simulink model "vippip_win"  (Simulink 6.4)
settings: Solver=FixedStepDiscrete  StartTime=0.0  StopTime=inf  RelTol=1e-3
InitFcn:
  | initChan = str2num(get_param([bdroot(gcs) '/Control'],'pip_ch'));
model workspace: external: M-Code (data not in the file)
libraries: simulink x4, dspsigops x4, dspwin32 x3, vipgeotforms x2, dspswit3 x2, dspbuff3 x2, vipmisc x1, viptextngfix x1, vipsnks x1
CloseFcn:
  | clear initChan
settings Model: Creator=asharma  LastModifiedBy=Pr . Saddam&Ali
settings DataIOCC: SaveOutput=off  SaveTime=off
settings OptimizationCC: InlineInvariantSignals=on
settings DebuggingCC: StrictBusMsg=None

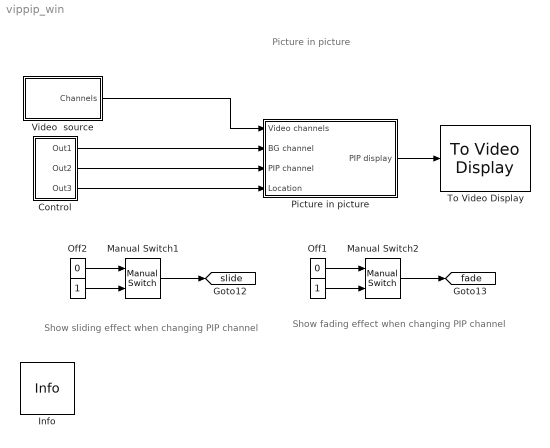
== system vippip_win ==
  note: Picture in picture
  note: Show sliding effect when
      | changing PIP channel
  note: Show fading effect  when
      |  changing PIP channel
  " " : Constant  Value=1  OutDataTypeMode=boolean  OutDataType=sfix(16)  ConRadixGroup=Use specified scaling  OutScaling=2^0  SampleTime=inf  FramePeriod=inf
  "   " : Constant  Value=1  OutDataTypeMode=boolean  OutDataType=sfix(16)  ConRadixGroup=Use specified scaling  OutScaling=2^0  SampleTime=inf  FramePeriod=inf
  Control : Subsystem  mask(Control){main_ch=1, pip_ch=2, piplocation=Lower left}
      mask prompts: main_ch "Main channel number"; pip_ch "PIP channel number"; piplocation "Location of PIP window"
      mask help: User this mask to control the channel choices and location of the picture in picture (PIP) window.
      mask init:
      | if (piplocation==1)
      |     quadLoc1= '[0 0]';
      | elseif (piplocation==2)
      |     quadLoc1 = '[0 80]';
      | elseif (piplocation==4)
      |     quadLoc1= '[60 80]';
      | else
      |     quadLoc1 = '[60 0]';
      | end
      | set_param([gcb '/Location of PIP video'], 'Value', quadLoc1);
      mask StyleString: popup(1|2|3),popup(1|2|3),popup(Upper left|Upper right|Lower left|Lower right)
      mask Display: disp('Control');
  Info : vipmisc/Info  SystemSampleTime=-1
  Manual Switch1 : simulink/Signal Routing/Manual Switch  SystemSampleTime=-1  sw=0  action=0
  Manual Switch2 : simulink/Signal Routing/Manual Switch  SystemSampleTime=-1  sw=0  action=0
  Off1 : Constant  Value=0  OutDataTypeMode=boolean  OutDataType=sfix(16)  ConRadixGroup=Use specified scaling  OutScaling=2^0  SampleTime=inf  FramePeriod=inf
  Off2 : Constant  Value=0  OutDataTypeMode=boolean  OutDataType=sfix(16)  ConRadixGroup=Use specified scaling  OutScaling=2^0  SampleTime=inf  FramePeriod=inf
  Picture in picture : Subsystem
  To Video Display : vipsnks/To Video Display  inputType=Intensity  OutputDevice=On-screen video monitor  fullScreen=off  videoWindowX=711  videoWindowY=334  saveWindowSize=off  videoWindowWidth=168  videoWindowHeight=147
  Video  source : Subsystem
  tag scope: fade=global, slide=global
  wires:
  Picture in picture/1(PIP display) -> To Video Display/1
  Off1/1 -> Manual Switch2/1
  "   "/1 -> Manual Switch2/2
  Manual Switch2/1 -> [fade]
  Off2/1 -> Manual Switch1/1
  " "/1 -> Manual Switch1/2
  Manual Switch1/1 -> [slide]
  Video  source/1(Channels) -> Picture in picture/1(Video channels)
  Control/1(Out1) -> Picture in picture/2(BG channel)
  Control/2(Out2) -> Picture in picture/3(PIP channel)
  Control/3(Out3) -> Picture in picture/4(Location)

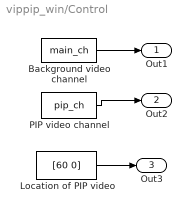
== system vippip_win/Control ==
  Background video channel : Constant  Value=main_ch  OutDataTypeMode=single  OutDataType=sfix(16)  ConRadixGroup=Use specified scaling  OutScaling=2^0  SampleTime=1/30  FramePeriod=inf
  Location of PIP video : Constant  Value=[60 0]  OutDataTypeMode=single  OutDataType=sfix(16)  ConRadixGroup=Use specified scaling  OutScaling=2^0  SampleTime=1/30  FramePeriod=inf
  PIP video channel : Constant  Value=pip_ch  OutDataTypeMode=single  OutDataType=sfix(16)  ConRadixGroup=Use specified scaling  OutScaling=2^0  SampleTime=1/30  FramePeriod=inf
  Out1 : Outport
  Out2 : Outport  Port=2
  Out3 : Outport  Port=3
  wires:
  Background video channel/1 -> Out1/1
  PIP video channel/1 -> Out2/1
  Location of PIP video/1 -> Out3/1

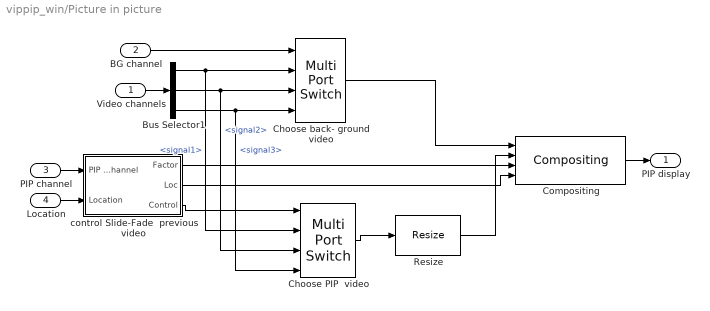
== system vippip_win/Picture in picture ==
  Video channels : Inport
  BG channel : Inport  Port=2
  PIP channel : Inport  Port=3
  Location : Inport  Port=4
  Bus Selector1 : BusSelector  OutputSignals=signal1,signal2,signal3
  Choose PIP  video : MultiPortSwitch  Inputs=3  InputSameDT=on
  Choose back- ground video : MultiPortSwitch  Inputs=3  InputSameDT=on
  Compositing : viptextngfix/Compositing  DialogController=vipDDGCreate  DialogControllerArgs=DataTag0  operation=Blend  bFacSrc=Input port  mFacSrc=Specify via dialog  bFactor=0.5  mFactor=1  source=Input port  coordinates=[0 0]  prodOutputMode=Binary point scaling  prodOutputWordLength=32  prodOutputFracLength=10  roundingMode=Floor  overflowMode=off
  Resize : vipgeotforms/Resize  DialogController=vipDDGCreate  DialogControllerArgs=DataTag1  specify=Output size as a percentage of input size  rfactor=50  outCols=25  outRows=25  outRowsCols=[60 80]  interp_method=Bilinear  antialias=on  prodOutputMode=Binary point scaling  prodOutputWordLength=32  prodOutputFracLength=10  roundingMode=Nearest  overflowMode=on
  control Slide-Fade  previous video : Subsystem
  PIP display : Outport
  wires:
  Choose PIP  video/1 -> Resize/1
  control Slide-Fade  previous video/3(Control) -> Choose PIP  video/1
  control Slide-Fade  previous video/2(Loc) -> Compositing/4
  control Slide-Fade  previous video/1(Factor) -> Compositing/3
  Choose back- ground video/1 -> Compositing/1
  Resize/1 -> Compositing/2
  Bus Selector1/1 -> Choose back- ground video/2, Choose PIP  video/2  "<signal1>"
  Bus Selector1/2 -> Choose back- ground video/3, Choose PIP  video/3  "<signal2>"
  Bus Selector1/3 -> Choose back- ground video/4, Choose PIP  video/4  "<signal3>"
  BG channel/1 -> Choose back- ground video/1
  Video channels/1 -> Bus Selector1/1
  Compositing/1 -> PIP display/1
  PIP channel/1 -> control Slide-Fade  previous video/1(PIP video channel)
  Location/1 -> control Slide-Fade  previous video/2(Location)

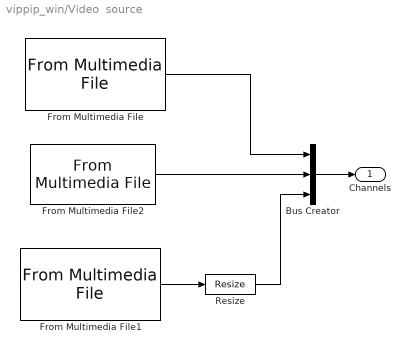
== system vippip_win/Video  source ==
  Bus Creator : BusCreator  Inputs=3
  From Multimedia File : dspwin32/From Multimedia File  DialogController=dspDDGCreate  DialogControllerArgs=DataTag2  inputFilename=cat_video.avi  loop=on  numPlays=inf  outputStreams=Video and audio  videoDataType=single  audioDataType=int16  inheritSampleTime=on  userDefinedSampleTime=1/30  noAudioOutput=off  isIntensityVideo=on  outputEOF=off
  From Multimedia File1 : dspwin32/From Multimedia File  DialogController=dspDDGCreate  DialogControllerArgs=DataTag3  inputFilename=shaky_car.avi  loop=on  numPlays=inf  outputStreams=Video and audio  videoDataType=single  audioDataType=int16  inheritSampleTime=on  userDefinedSampleTime=1/30  noAudioOutput=off  isIntensityVideo=on  outputEOF=off
  From Multimedia File2 : dspwin32/From Multimedia File  DialogController=dspDDGCreate  DialogControllerArgs=DataTag4  inputFilename=vipmen.avi  loop=on  numPlays=inf  outputStreams=Video and audio  videoDataType=single  audioDataType=int16  inheritSampleTime=on  userDefinedSampleTime=1/30  noAudioOutput=off  isIntensityVideo=on  outputEOF=off
  Resize : vipgeotforms/Resize  DialogController=vipDDGCreate  DialogControllerArgs=DataTag5  specify=Number of output rows and columns  rfactor=200  outCols=25  outRows=25  outRowsCols=[120 160]  interp_method=Bilinear  antialias=on  prodOutputMode=Binary point scaling  prodOutputWordLength=32  prodOutputFracLength=10  roundingMode=Nearest  overflowMode=on
  Channels : Outport
  wires:
  From Multimedia File1/1 -> Resize/1
  From Multimedia File/1 -> Bus Creator/1
  From Multimedia File2/1 -> Bus Creator/2
  Resize/1 -> Bus Creator/3
  Bus Creator/1 -> Channels/1

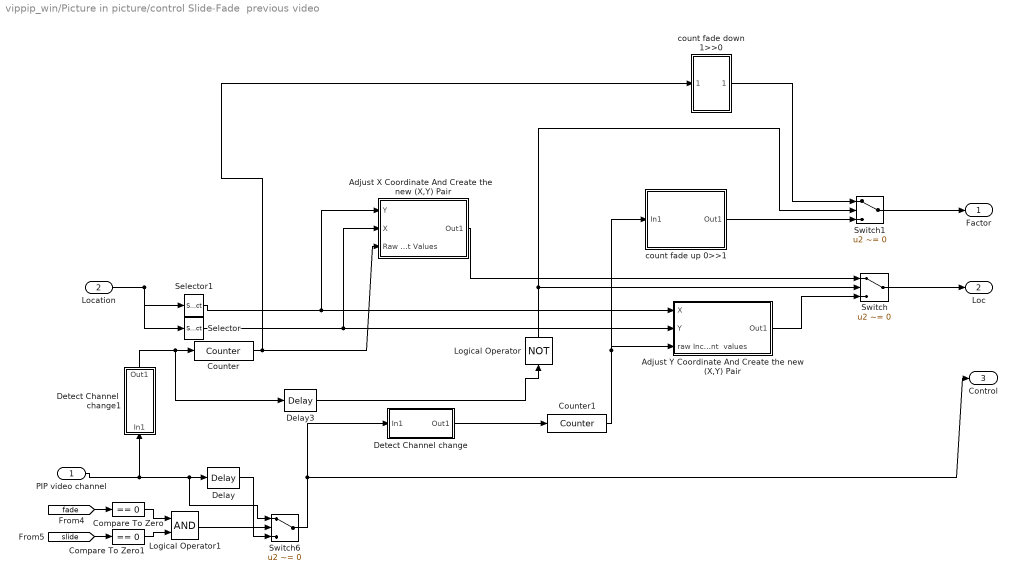
== system vippip_win/Picture in picture/control Slide-Fade  previous video ==
  PIP video channel : Inport
  Location : Inport  Port=2
  Adjust X Coordinate And Create the   new (X,Y) Pair : Subsystem
  Adjust Y Coordinate And Create the new (X,Y) Pair : Subsystem
  Compare To Zero : simulink/Logic and Bit Operations/Compare To Zero  SystemSampleTime=-1  relop===  LogicOutDataTypeMode=uint8  ZeroCross=off
  Compare To Zero1 : simulink/Logic and Bit Operations/Compare To Zero  SystemSampleTime=-1  relop===  LogicOutDataTypeMode=uint8  ZeroCross=off
  Counter : dspswit3/Counter  Direction=Up  CountEvent=Non-zero sample  CounterSize=User defined  MaxCount=31  InitialCount=0  Output=Count  HitValue=32  ResetInput=off  SamplesPerFrame=1  Ts=1/(30.0375)  CntDtype=single  HitDtype=Logical
  Counter1 : dspswit3/Counter  Direction=Up  CountEvent=Non-zero sample  CounterSize=User defined  MaxCount=31  InitialCount=0  Output=Count  HitValue=32  ResetInput=off  SamplesPerFrame=1  Ts=1/(30.0375)  CntDtype=single  HitDtype=Logical
  Delay : dspsigops/Delay  dly_unit=Samples  delay=32  ic_detail=on  dif_ic_for_ch=off  dif_ic_for_dly=off  ic=initChan  reset_popup=None
  Delay3 : dspsigops/Delay  dly_unit=Samples  delay=31  ic_detail=on  dif_ic_for_ch=off  dif_ic_for_dly=off  ic=initChan  reset_popup=None
  Detect Channel  change1 : Subsystem  Orientation=up
  Detect Channel change : Subsystem
  Logical Operator : Logic  Orientation=up  Operator=NOT  AllPortsSameDT=off  OutDataTypeMode=Boolean
  Logical Operator1 : Logic  AllPortsSameDT=off  OutDataTypeMode=Boolean
  Selector : Selector  Elements=2  InputPortWidth=2
  Selector1 : Selector  InputPortWidth=2
  Switch : Switch  Criteria=u2 ~= 0
  Switch1 : Switch  Criteria=u2 ~= 0
  Switch6 : Switch  Criteria=u2 ~= 0
  count fade down 1>>0 : Subsystem
  count fade up 0>>1 : Subsystem
  Factor : Outport
  Loc : Outport  Port=2
  Control : Outport  Port=3
  wires:
  Switch6/1 -> Control/1, Detect Channel change/1(In1)
  Delay/1 -> Switch6/3
  Logical Operator1/1 -> Switch6/2
  Compare To Zero1/1 -> Logical Operator1/2
  Compare To Zero/1 -> Logical Operator1/1
  [slide] -> Compare To Zero1/1
  [fade] -> Compare To Zero/1
  count fade up 0>>1/1(Out1) -> Switch1/3
  PIP video channel/1 -> Switch6/1, Delay/1, Detect Channel  change1/1(In1)
  Counter/1 -> count fade down 1>>0/1(In1), Adjust X Coordinate And Create the   new (X,Y) Pair/3(Raw Count Values)
  Selector1/1 -> Adjust Y Coordinate And Create the new (X,Y) Pair/1(X), Adjust X Coordinate And Create the   new (X,Y) Pair/1(Y)
  Location/1 -> Selector/1, Selector1/1
  Selector/1 -> Adjust Y Coordinate And Create the new (X,Y) Pair/2(Y), Adjust X Coordinate And Create the   new (X,Y) Pair/2(X)
  Detect Channel  change1/1(Out1) -> Counter/1, Delay3/1
  Detect Channel change/1(Out1) -> Counter1/1
  Counter1/1 -> count fade up 0>>1/1(In1), Adjust Y Coordinate And Create the new (X,Y) Pair/3(raw Increment  values)
  Adjust X Coordinate And Create the   new (X,Y) Pair/1(Out1) -> Switch/1
  Adjust Y Coordinate And Create the new (X,Y) Pair/1(Out1) -> Switch/3
  Switch/1 -> Loc/1
  Logical Operator/1 -> Switch/2, Switch1/2
  Delay3/1 -> Logical Operator/1
  count fade down 1>>0/1(Out1) -> Switch1/1
  Switch1/1 -> Factor/1

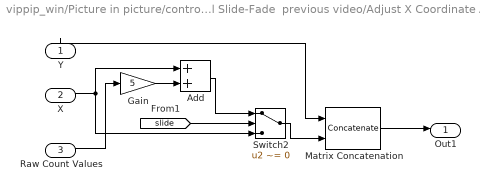
== system vippip_win/Picture in picture/control Slide-Fade  previous video/Adjust X Coordinate And Create the   new (X,Y) Pair ==
  Y : Inport  Orientation=up
  X : Inport  Port=2
  Raw Count Values : Inport  Port=3
  Add : Sum  OutScaling=2^-10
  Gain : Gain  Gain=5
  Matrix Concatenation : Concatenate  Mode=Horizontal matrix concatenation
  Switch2 : Switch  Criteria=u2 ~= 0
  Out1 : Outport
  wires:
  Switch2/1 -> Matrix Concatenation/2
  Add/1 -> Switch2/1
  [slide] -> Switch2/2
  Gain/1 -> Add/2
  Y/1 -> Matrix Concatenation/1
  X/1 -> Add/1, Switch2/3
  Raw Count Values/1 -> Gain/1
  Matrix Concatenation/1 -> Out1/1

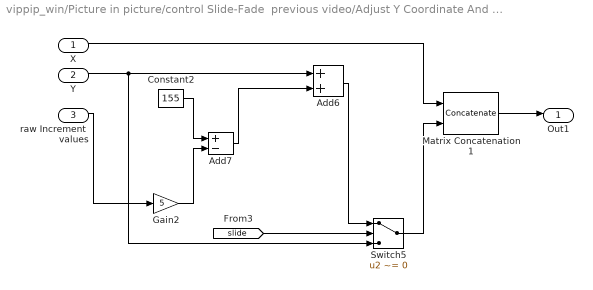
== system vippip_win/Picture in picture/control Slide-Fade  previous video/Adjust Y Coordinate And Create the new (X,Y) Pair ==
  X : Inport
  Y : Inport  Port=2
  raw Increment  values : Inport  Port=3
  Add6 : Sum  OutScaling=2^-10
  Add7 : Sum  Inputs=+-  OutScaling=2^-10
  Constant2 : Constant  Value=155  OutDataTypeMode=single  OutDataType=sfix(16)  ConRadixGroup=Use specified scaling  OutScaling=2^0  SampleTime=1/30  FramePeriod=inf
  Gain2 : Gain  Gain=5
  Matrix Concatenation1 : Concatenate  Mode=Horizontal matrix concatenation
  Switch5 : Switch  Criteria=u2 ~= 0
  Out1 : Outport
  wires:
  Switch5/1 -> Matrix Concatenation1/2
  Add6/1 -> Switch5/1
  [slide] -> Switch5/2
  Gain2/1 -> Add7/2
  Add7/1 -> Add6/2
  Constant2/1 -> Add7/1
  X/1 -> Matrix Concatenation1/1
  Y/1 -> Switch5/3, Add6/1
  raw Increment  values/1 -> Gain2/1
  Matrix Concatenation1/1 -> Out1/1

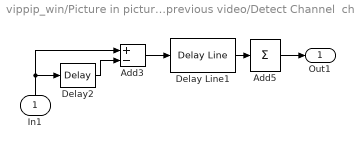
== system vippip_win/Picture in picture/control Slide-Fade  previous video/Detect Channel  change1 ==
  In1 : Inport  Orientation=up
  Add3 : Sum  Inputs=+-  OutScaling=2^-10
  Add5 : Sum  Inputs=+  OutScaling=2^-10
  Delay Line1 : dspbuff3/Delay Line  siz=32  ic=0  directfeed=off
  Delay2 : dspsigops/Delay  dly_unit=Samples  delay=1  ic_detail=on  dif_ic_for_ch=off  dif_ic_for_dly=off  ic=initChan  reset_popup=None
  Out1 : Outport
  wires:
  Add5/1 -> Out1/1
  In1/1 -> Delay2/1, Add3/1
  Delay Line1/1 -> Add5/1
  Add3/1 -> Delay Line1/1
  Delay2/1 -> Add3/2

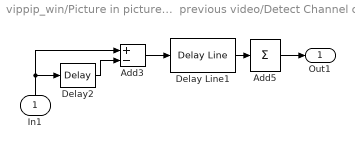
== system vippip_win/Picture in picture/control Slide-Fade  previous video/Detect Channel change ==
  In1 : Inport  Orientation=up
  Add3 : Sum  Inputs=+-  OutScaling=2^-10
  Add5 : Sum  Inputs=+  OutScaling=2^-10
  Delay Line1 : dspbuff3/Delay Line  siz=32  ic=0  directfeed=off
  Delay2 : dspsigops/Delay  dly_unit=Samples  delay=1  ic_detail=on  dif_ic_for_ch=off  dif_ic_for_dly=off  ic=0  reset_popup=None
  Out1 : Outport
  wires:
  Delay2/1 -> Add3/2
  Add3/1 -> Delay Line1/1
  Delay Line1/1 -> Add5/1
  In1/1 -> Add3/1, Delay2/1
  Add5/1 -> Out1/1

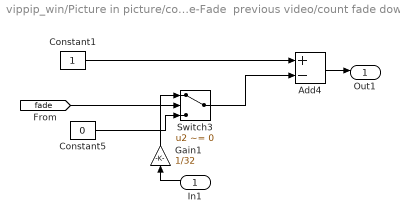
== system vippip_win/Picture in picture/control Slide-Fade  previous video/count fade down 1>>0 ==
  In1 : Inport  Orientation=left
  Add4 : Sum  Inputs=+-  OutScaling=2^-10
  Constant1 : Constant  Value=1  OutDataTypeMode=single  OutDataType=sfix(16)  ConRadixGroup=Use specified scaling  OutScaling=2^0  SampleTime=1/30  FramePeriod=inf
  Constant5 : Constant  Value=0  OutDataTypeMode=single  OutDataType=sfix(16)  ConRadixGroup=Use specified scaling  OutScaling=2^0  SampleTime=1/30  FramePeriod=inf
  Gain1 : Gain  Orientation=up  Gain=1/32
  Switch3 : Switch  Criteria=u2 ~= 0
  Out1 : Outport
  wires:
  Constant5/1 -> Switch3/3
  Switch3/1 -> Add4/2
  Gain1/1 -> Switch3/1
  [fade] -> Switch3/2
  Constant1/1 -> Add4/1
  In1/1 -> Gain1/1
  Add4/1 -> Out1/1

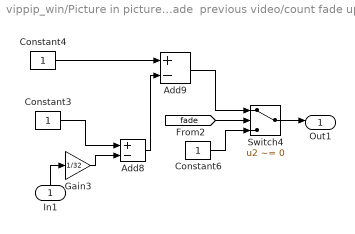
== system vippip_win/Picture in picture/control Slide-Fade  previous video/count fade up 0>>1 ==
  In1 : Inport  Orientation=up
  Add8 : Sum  Inputs=+-  OutScaling=2^-10
  Add9 : Sum  Inputs=+-  OutScaling=2^-10
  Constant3 : Constant  Value=1  OutDataTypeMode=single  OutDataType=sfix(16)  ConRadixGroup=Use specified scaling  OutScaling=2^0  SampleTime=1/30  FramePeriod=inf
  Constant4 : Constant  Value=1  OutDataTypeMode=single  OutDataType=sfix(16)  ConRadixGroup=Use specified scaling  OutScaling=2^0  SampleTime=1/30  FramePeriod=inf
  Constant6 : Constant  Value=1  OutDataTypeMode=single  OutDataType=sfix(16)  ConRadixGroup=Use specified scaling  OutScaling=2^0  SampleTime=1/30  FramePeriod=inf
  Gain3 : Gain  Gain=1/32
  Switch4 : Switch  Criteria=u2 ~= 0
  Out1 : Outport
  wires:
  Constant6/1 -> Switch4/3
  Add9/1 -> Switch4/1
  [fade] -> Switch4/2
  Constant3/1 -> Add8/1
  Gain3/1 -> Add8/2
  Add8/1 -> Add9/2
  Constant4/1 -> Add9/1
  In1/1 -> Gain3/1
  Switch4/1 -> Out1/1
